simulink model "bareSystem"  (R2013b)
settings: Solver=ode1  StartTime=0.0  StopTime=tSim  FixedStep=0.1  RelTol=1e-3
values from neighbouring files (symbols this model uses):
  initial_state = -1    [launcher.m]
  input = 1    [launcher.m]
  k = 4    [launcher.m]
  T = 3    [launcher.m]
settings Model: Creator=JT  LastModifiedBy=JT

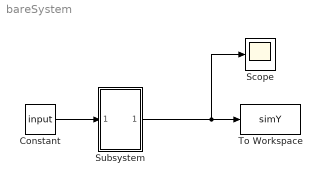
== system bareSystem ==
  Constant : Constant  Value=input
  Scope : Scope
  Subsystem : Subsystem
  To Workspace : ToWorkspace  VariableName=simY  SampleTime=-1
  wires:
  Constant/1 -> Subsystem/1(In1)
  Subsystem/1(Out1) -> Scope/1, To Workspace/1

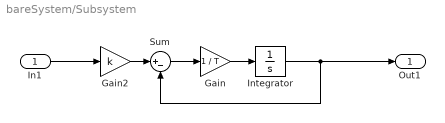
== system bareSystem/Subsystem ==
  In1 : Inport
  Gain : Gain  Gain=1 / T
  Gain2 : Gain  Gain=k
  Integrator : Integrator  InitialCondition=initial_state
  Sum : Sum  Inputs=|+-
  Out1 : Outport
  wires:
  Sum/1 -> Gain/1
  Integrator/1 -> Out1/1, Sum/2
  Gain2/1 -> Sum/1
  In1/1 -> Gain2/1
  Gain/1 -> Integrator/1
